simulink model "speedcontrol_dcmotor"  (R2014a)
settings: Solver=FixedStepDiscrete  StartTime=0.0  StopTime=10  FixedStep=Ts  RelTol=1e-3
PreLoadFcn:
  | warning('off','ne_sli:simulator:linearize:LocalSolverLinearizationUnsupported');
  | Ts = 1e-3;
  | Tc1 = 1e-3;
  | Tc2 = 1e-3;
libraries: fl_lib x13, nesl_utility x7, simulink x4, elec_lib x3
settings Model: Creator=mcuenant  LastModifiedBy=cosorio
settings DataIOCC: LimitDataPoints=off  SaveOutput=off  DSMLogging=off  SaveTime=off  SignalLoggingName=DCMotorDataLog
settings OptimizationCC: OptimizeModelRefInitCode=on
settings DebuggingCC: AlgebraicLoopMsg=error  UnderspecifiedInitializationDetection=Classic  SolverPrmCheckMsg=none  StateNameClashWarn=warning
settings RTWCC: SystemTargetFile=ert.tlc  GenCodeOnly=on  TemplateMakefile=ert_default_tmf  Description=Embedded Coder  GenerateReport=on  ProcessScript=ert_make_rtw_hook  IncludeHyperlinkInReport=on  LaunchReport=on  GenerateTraceInfo=on  GenerateWebview=on  GenerateCodeMetricsReport=on
settings CodeAppCC: IgnoreCustomStorageClasses=off  SimulinkDataObjDesc=on  SFDataObjDesc=on  InsertBlockDesc=on  ReqsInCode=on
settings ERTTargetCC: ParMdlRefBuildCompliant=on  CompOptLevelCompliant=on  ConcurrentExecutionCompliant=on  ERTFirstTimeCompliant=on  ModelStepFunctionPrototypeControlCompliant=on  CPPClassGenCompliant=on  ERTCustomFileTemplate=example_file_process.tlc

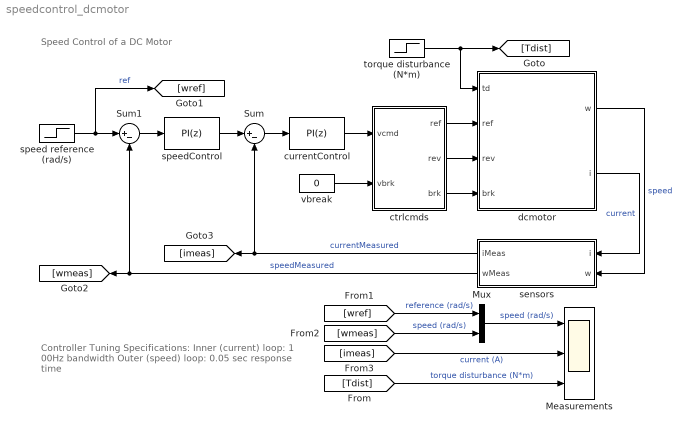
== system speedcontrol_dcmotor ==
  note: Controller Tuning Specifications:
      | Inner (current) loop: 1 00Hz bandwidth
      | Outer (speed) loop: 0.05 sec response time
  note: Speed Control of a DC Motor
  Measurements : Scope  NumInputPorts=3
      settings: YMin=-0.2~-10~-0.4  YMax=1.2~10~0.4  SaveName=DCMotorData
  Mux : Mux  Inputs=2
  Sum : Sum  Inputs=|+-
  Sum1 : Sum  Inputs=|+-
  ctrlcmds : Subsystem
  currentControl : simulink/Continuous/PID Controller  Controller=PI  TimeDomain=Discrete-time  SampleTime=Tc2  IntegratorMethod=Forward Euler  FilterMethod=Forward Euler  Form=Parallel  P=1  I=1  D=0  N=100  InitialConditionSource=internal  InitialConditionForIntegrator=0  InitialConditionForFilter=0  ExternalReset=none  LimitOutput=off  UpperSaturationLimit=inf  LowerSaturationLimit=-inf  LinearizeAsGain=off  AntiWindupMode=none  Kb=1  TrackingMode=off  Kt=1  PParamMin=[]  PParamMax=[]  IParamMin=[]  IParamMax=[]  DParamMin=[]  DParamMax=[]  NParamMin=[]  NParamMax=[]  KbParamMin=[]  KbParamMax=[]  KtParamMin=[]  KtParamMax=[]  POutMin=[]  POutMax=[]  IOutMin=[]  IOutMax=[]  DOutMin=[]  DOutMax=[]  NOutMin=[]  NOutMax=[]  KbOutMin=[]  KbOutMax=[]  KtOutMin=[]  KtOutMax=[]  IntegratorOutMin=[]  IntegratorOutMax=[]  FilterOutMin=[]  FilterOutMax=[]  SumOutMin=[]  SumOutMax=[]  SumI1OutMin=[]  SumI1OutMax=[]  SumI2OutMin=[]  SumI2OutMax=[]  SumI3OutMin=[]  SumI3OutMax=[]  SumDOutMin=[]  SumDOutMax=[]  SaturationOutMin=[]  SaturationOutMax=[]  IntegratorContinuousStateAttributes=''  IntegratorStateMustResolveToSignalObject=off  IntegratorRTWStateStorageClass=Auto  FilterContinuousStateAttributes=''  FilterStateMustResolveToSignalObject=off  FilterRTWStateStorageClass=Auto
  dcmotor : Subsystem
  sensors : Subsystem
  speed reference (rad/s) : Step  Time=2  SampleTime=Tc1
  speedControl : simulink/Continuous/PID Controller  Controller=PI  TimeDomain=Discrete-time  SampleTime=Tc1  IntegratorMethod=Forward Euler  FilterMethod=Forward Euler  Form=Parallel  P=1  I=1  D=0  N=100  InitialConditionSource=internal  InitialConditionForIntegrator=0  InitialConditionForFilter=0  ExternalReset=none  LimitOutput=off  UpperSaturationLimit=inf  LowerSaturationLimit=-inf  LinearizeAsGain=off  AntiWindupMode=none  Kb=1  TrackingMode=off  Kt=1  PParamMin=[]  PParamMax=[]  IParamMin=[]  IParamMax=[]  DParamMin=[]  DParamMax=[]  NParamMin=[]  NParamMax=[]  KbParamMin=[]  KbParamMax=[]  KtParamMin=[]  KtParamMax=[]  POutMin=[]  POutMax=[]  IOutMin=[]  IOutMax=[]  DOutMin=[]  DOutMax=[]  NOutMin=[]  NOutMax=[]  KbOutMin=[]  KbOutMax=[]  KtOutMin=[]  KtOutMax=[]  IntegratorOutMin=[]  IntegratorOutMax=[]  FilterOutMin=[]  FilterOutMax=[]  SumOutMin=[]  SumOutMax=[]  SumI1OutMin=[]  SumI1OutMax=[]  SumI2OutMin=[]  SumI2OutMax=[]  SumI3OutMin=[]  SumI3OutMax=[]  SumDOutMin=[]  SumDOutMax=[]  SaturationOutMin=[]  SaturationOutMax=[]  IntegratorContinuousStateAttributes=''  IntegratorStateMustResolveToSignalObject=off  IntegratorRTWStateStorageClass=Auto  FilterContinuousStateAttributes=''  FilterStateMustResolveToSignalObject=off  FilterRTWStateStorageClass=Auto
  "torque disturbance (N*m) " : Step  Time=6  After=-0.2  SampleTime=Ts
  vbreak : Constant  Value=0  SampleTime=Tc2
  wires:
  dcmotor/2(i) -> sensors/1(i)  "current"
  dcmotor/1(w) -> sensors/2(w)  "speed"
  "torque disturbance (N*m) "/1 -> [Tdist], dcmotor/1(td)
  Sum/1 -> currentControl/1
  sensors/2(wMeas) -> [wmeas], Sum1/2  "speedMeasured"
  Sum1/1 -> speedControl/1
  sensors/1(iMeas) -> Sum/2, [imeas]  "currentMeasured"
  speedControl/1 -> Sum/1
  speed reference (rad/s)/1 -> Sum1/1, [wref]  "ref"
  [wref] -> Mux/1  "reference (rad/s)"
  [wmeas] -> Mux/2  "speed (rad/s)"
  Mux/1 -> Measurements/1  "speed (rad/s)"
  currentControl/1 -> ctrlcmds/1(vcmd)
  vbreak/1 -> ctrlcmds/2(vbrk)
  ctrlcmds/1(ref) -> dcmotor/2(ref)
  ctrlcmds/2(rev) -> dcmotor/3(rev)
  ctrlcmds/3(brk) -> dcmotor/4(brk)
  [Tdist] -> Measurements/3  "torque disturbance (N*m)"
  [imeas] -> Measurements/2  "current (A)"

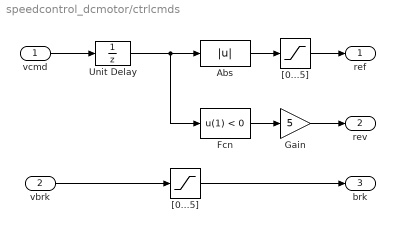
== system speedcontrol_dcmotor/ctrlcmds ==
  vcmd : Inport
  vbrk : Inport  Port=2
  Abs : Abs
  Fcn : Fcn  Expr=u(1) < 0
  Gain : Gain  Gain=5
  Unit Delay : UnitDelay  SampleTime=Tc2
  "[0...5]" : Saturate  UpperLimit=5  LowerLimit=0
  "[0...5] " : Saturate  UpperLimit=5  LowerLimit=0
  ref : Outport
  rev : Outport  Port=2
  brk : Outport  Port=3
  wires:
  "[0...5] "/1 -> brk/1
  vbrk/1 -> "[0...5] "/1
  Abs/1 -> "[0...5]"/1
  Fcn/1 -> Gain/1
  "[0...5]"/1 -> ref/1
  Gain/1 -> rev/1
  vcmd/1 -> Unit Delay/1
  Unit Delay/1 -> Fcn/1, Abs/1

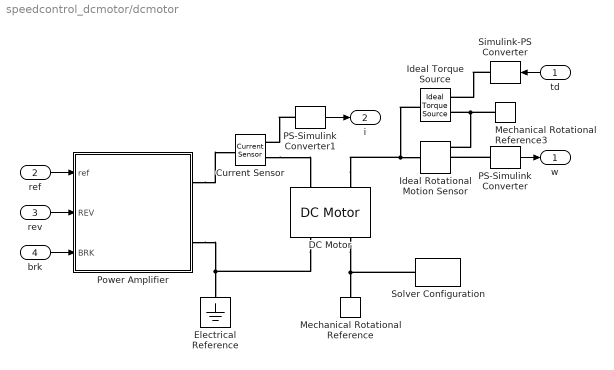
== system speedcontrol_dcmotor/dcmotor ==
  td : Inport
  ref : Inport  Port=2
  rev : Inport  Port=3
  brk : Inport  Port=4
  Current Sensor : fl_lib/Electrical/Electrical Sensors/Current Sensor
  DC Motor : elec_lib/Actuators & Drivers/Rotational Actuators/DC Motor  parameterization=1  Ra=4 Ohm  La=2e-6 H  emf_or_torque=1  Kv=0.3 V/(rad/s)  Ki=6.876e-4 N*m/A  T_stall=2.4e-4 N*m  w_max=1.91e+4 rpm  w_rated=1.5e+4 rpm  P_rated=0.08 W  V_rated=1.5 V  J=0.01 kg*m^2  lam_param=1  lam=1 N*m/(rad/s)  i_noload=0 A  V_i_noload=1.5 V  speed0=0 rpm  alpha=0.00393 1/K  Tmeas=25 C  thermal_mass=100 J/K  initial_temperature=25 C
  Electrical Reference : fl_lib/Electrical/Electrical Elements/Electrical Reference
  Ideal Torque Source : fl_lib/Mechanical/Mechanical Sources/Ideal Torque Source
  Ideal Rotational Motion Sensor : fl_lib/Mechanical/Mechanical Sensors/Ideal Rotational Motion Sensor  offset=0 rad
  Mechanical Rotational Reference : fl_lib/Mechanical/Rotational Elements/Mechanical Rotational Reference
  Mechanical Rotational Reference3 : fl_lib/Mechanical/Rotational Elements/Mechanical Rotational Reference
  PS-Simulink Converter : nesl_utility/PS-Simulink Converter  PhysicalDomain=network_engine_domain  SubClassName=ps_output  LeftPortType=input  RightPortType=output  PseudoPeriodic=off  Frequencies=[]  Unit=rad/s  AffineConversion=off
  PS-Simulink Converter1 : nesl_utility/PS-Simulink Converter  PhysicalDomain=network_engine_domain  SubClassName=ps_output  LeftPortType=input  RightPortType=output  PseudoPeriodic=off  Frequencies=[]  Unit=A  AffineConversion=off
  Power Amplifier : Subsystem
  Simulink-PS Converter : nesl_utility/Simulink-PS Converter  PhysicalDomain=network_engine_domain  SubClassName=ps_input  LeftPortType=input  RightPortType=output  PseudoPeriodic=off  Frequencies=[]  NoiseDistribution=none  NoiseParameters=[]  Unit=N*m  AffineConversion=off  InputFiltering=off  SimscapeFilterOrder=1  InputFilterTimeConstant=.001  UdotUserProvided=1
  Solver Configuration : nesl_utility/Solver Configuration  PhysicalDomain=network_engine_domain  SubClassName=solver  LeftPortType=input  RightPortType=generic  Accelerate=off  Tones=[]  Harmonics=[]  SimulateNoise=off  Profile=off  UseLocalSampling=off  EnableSwitchedLinearOptims=on  FrequencyDomain=off  UseCCode=off  RelTol=0.001  AbsTol=1e-06  MinStep=1e-09  ToWorkspace=off  DoDC=off  ResidualTolerance=1e-9  UseLocalSolver=on  LocalSolverChoice=NE_BACKWARD_EULER_ADVANCER  LocalSolverSampleTime=Ts  DoFixedCost=on  MaxNonlinIter=6  MaxModeIter=2  LinearAlgebra=Sparse  DelaysMemoryBudget=1024  AutomaticFiltering=off  FilteringTimeConstant=0.001
  w : Outport
  i : Outport  Port=2
  wires:
  PS-Simulink Converter/1 -> w/1
  PS-Simulink Converter1/1 -> i/1
  td/1 -> Simulink-PS Converter/1
  ref/1 -> Power Amplifier/1(ref)
  rev/1 -> Power Amplifier/2(REV)
  brk/1 -> Power Amplifier/3(BRK)
  connections:
  DC Motor/RConn1 -- Power Amplifier/RConn2 -- Electrical Reference/LConn1
  DC Motor/LConn2 -- Ideal Rotational Motion Sensor/LConn1 -- Ideal Torque Source/LConn1
  PS-Simulink Converter/LConn1 -- Ideal Rotational Motion Sensor/RConn2
  Simulink-PS Converter/RConn1 -- Ideal Torque Source/RConn1
  DC Motor/RConn2 -- Mechanical Rotational Reference/LConn1 -- Solver Configuration/RConn1
  PS-Simulink Converter1/LConn1 -- Current Sensor/RConn1
  Mechanical Rotational Reference3/LConn1 -- Ideal Rotational Motion Sensor/RConn1 -- Ideal Torque Source/RConn2
  Current Sensor/RConn2 -- DC Motor/LConn1
  Power Amplifier/RConn1 -- Current Sensor/LConn1

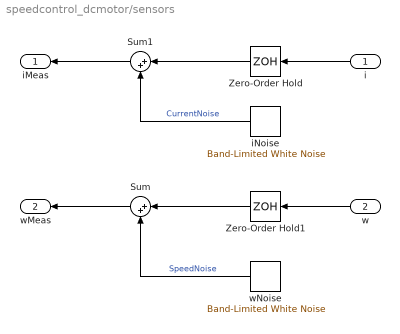
== system speedcontrol_dcmotor/sensors ==
  i : Inport
  w : Inport  Port=2
  Sum : Sum  Inputs=|++
  Sum1 : Sum  Inputs=|++
  Zero-Order Hold : ZeroOrderHold  SampleTime=Tc2
  Zero-Order Hold1 : ZeroOrderHold  SampleTime=Tc1
  iNoise : simulink/Sources/Band-Limited White Noise  Cov=(0.001)^2*Tc2*1  Ts=Tc2  seed=[23341]
  wNoise : simulink/Sources/Band-Limited White Noise  Cov=(0.01)^2*Tc1*1  Ts=Tc1  seed=[23341]
  iMeas : Outport
  wMeas : Outport  Port=2
  wires:
  w/1 -> Zero-Order Hold1/1
  i/1 -> Zero-Order Hold/1
  Zero-Order Hold1/1 -> Sum/1
  Zero-Order Hold/1 -> Sum1/1
  iNoise/1 -> Sum1/2  "CurrentNoise"
  wNoise/1 -> Sum/2  "SpeedNoise"
  Sum1/1 -> iMeas/1
  Sum/1 -> wMeas/1

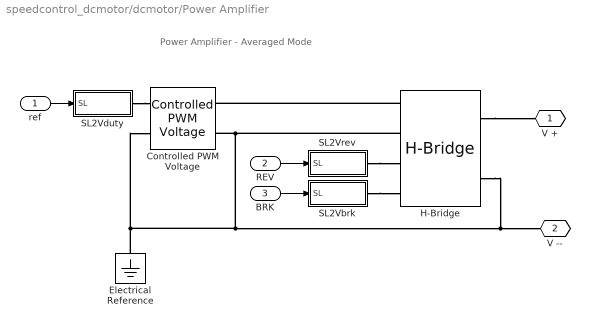
== system speedcontrol_dcmotor/dcmotor/Power Amplifier ==
  note: Power Amplifier - Averaged Mode
  ref : Inport
  REV : Inport  Port=2
  BRK : Inport  Port=3
  Controlled PWM Voltage : elec_lib/Actuators & Drivers/Drivers/Controlled PWM Voltage  F=1000 Hz  TD=0 s  pulse_width_offset=0 s  Vmin=0 V  Vmax=5 V  Vm=5 V  pwm_or_av=2  event_type=1  sample_time=1e-6 s
  Electrical Reference : fl_lib/Electrical/Electrical Elements/Electrical Reference
  H-Bridge : elec_lib/Actuators & Drivers/Drivers/H-Bridge  Venable=2.5 V  Vmax=5 V  Vreverse=2.5 V  Vbrake=2.5 V  Vm=30 V  pwm_or_av=2  discontinuous=0  freewheeling_mode=1  freewheeling_mode_disc=1  Ron=0.1 Ohm  Don=0.05 Ohm  Rload=10 Ohm  Lload=1e-5 H  F=10 kHz  w_vec=[1, 2] s  i_vec=[1, 2] A  vMatrix=[1, 2; 3, 4] V
  SL2Vbrk : Subsystem
  SL2Vduty : Subsystem
  SL2Vrev : Subsystem
  V + : PMIOPort  Tag=PMCPort  Port=1  Side=Right
  V -- : PMIOPort  Tag=PMCPort  Port=2  Side=Right
  wires:
  BRK/1 -> SL2Vbrk/1(SL)
  REV/1 -> SL2Vrev/1(SL)
  ref/1 -> SL2Vduty/1(SL)
  connections:
  SL2Vbrk/RConn1 -- H-Bridge/LConn4
  H-Bridge/LConn1 -- Controlled PWM Voltage/RConn1
  SL2Vduty/RConn1 -- Controlled PWM Voltage/LConn1
  H-Bridge/RConn1 -- V +/RConn1
  SL2Vrev/RConn1 -- H-Bridge/LConn3
  H-Bridge/LConn2 -- V --/RConn1 -- H-Bridge/RConn2 -- Electrical Reference/LConn1 -- Controlled PWM Voltage/LConn2 -- Controlled PWM Voltage/RConn2

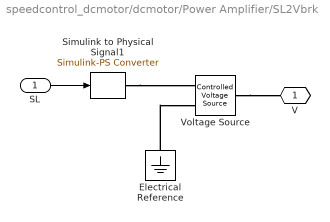
== system speedcontrol_dcmotor/dcmotor/Power Amplifier/SL2Vbrk ==
  SL : Inport
  Electrical Reference : fl_lib/Electrical/Electrical Elements/Electrical Reference
  Simulink to Physical Signal1 : nesl_utility/Simulink-PS Converter  PhysicalDomain=network_engine_domain  SubClassName=ps_input  LeftPortType=input  RightPortType=output  PseudoPeriodic=off  Frequencies=[]  NoiseDistribution=none  NoiseParameters=[]  Unit=V  AffineConversion=off  InputFiltering=off  SimscapeFilterOrder=1  InputFilterTimeConstant=.001  UdotUserProvided=1
  Voltage Source : fl_lib/Electrical/Electrical Sources/Controlled Voltage Source
  V : PMIOPort  Tag=PMCPort  Port=1  Side=Right
  wires:
  SL/1 -> Simulink to Physical Signal1/1
  connections:
  Electrical Reference/LConn1 -- Voltage Source/RConn2
  Simulink to Physical Signal1/RConn1 -- Voltage Source/RConn1
  Voltage Source/LConn1 -- V/RConn1

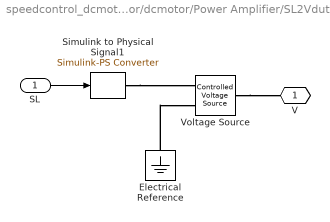
== system speedcontrol_dcmotor/dcmotor/Power Amplifier/SL2Vduty ==
  SL : Inport
  Electrical Reference : fl_lib/Electrical/Electrical Elements/Electrical Reference
  Simulink to Physical Signal1 : nesl_utility/Simulink-PS Converter  PhysicalDomain=network_engine_domain  SubClassName=ps_input  LeftPortType=input  RightPortType=output  PseudoPeriodic=off  Frequencies=[]  NoiseDistribution=none  NoiseParameters=[]  Unit=V  AffineConversion=off  InputFiltering=off  SimscapeFilterOrder=1  InputFilterTimeConstant=.001  UdotUserProvided=1
  Voltage Source : fl_lib/Electrical/Electrical Sources/Controlled Voltage Source
  V : PMIOPort  Tag=PMCPort  Port=1  Side=Right
  wires:
  SL/1 -> Simulink to Physical Signal1/1
  connections:
  Electrical Reference/LConn1 -- Voltage Source/RConn2
  Simulink to Physical Signal1/RConn1 -- Voltage Source/RConn1
  Voltage Source/LConn1 -- V/RConn1

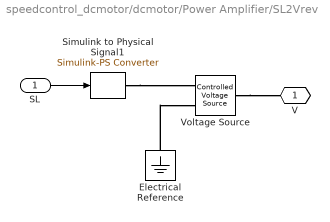
== system speedcontrol_dcmotor/dcmotor/Power Amplifier/SL2Vrev ==
  SL : Inport
  Electrical Reference : fl_lib/Electrical/Electrical Elements/Electrical Reference
  Simulink to Physical Signal1 : nesl_utility/Simulink-PS Converter  PhysicalDomain=network_engine_domain  SubClassName=ps_input  LeftPortType=input  RightPortType=output  PseudoPeriodic=off  Frequencies=[]  NoiseDistribution=none  NoiseParameters=[]  Unit=V  AffineConversion=off  InputFiltering=off  SimscapeFilterOrder=1  InputFilterTimeConstant=.001  UdotUserProvided=1
  Voltage Source : fl_lib/Electrical/Electrical Sources/Controlled Voltage Source
  V : PMIOPort  Tag=PMCPort  Port=1  Side=Right
  wires:
  SL/1 -> Simulink to Physical Signal1/1
  connections:
  Voltage Source/LConn1 -- V/RConn1
  Simulink to Physical Signal1/RConn1 -- Voltage Source/RConn1
  Electrical Reference/LConn1 -- Voltage Source/RConn2
